simulink model "neural_network_based_adaptive_sliding"  (R2020b)
settings: Solver=ode45  StartTime=0  StopTime=10  RelTol=1e-3
settings Model: Creator=Melik  LastModifiedBy=asus
settings DataIOCC: ReturnWorkspaceOutputs=off
settings DebuggingCC: ArithmeticOperatorsInVariantConditions=warning
settings SFSimCC: SimUseLocalCustomCode=off  CustomCodeUndefinedFunction=UseInterfaceOnly
settings RTWCC: RTWUseLocalCustomCode=off

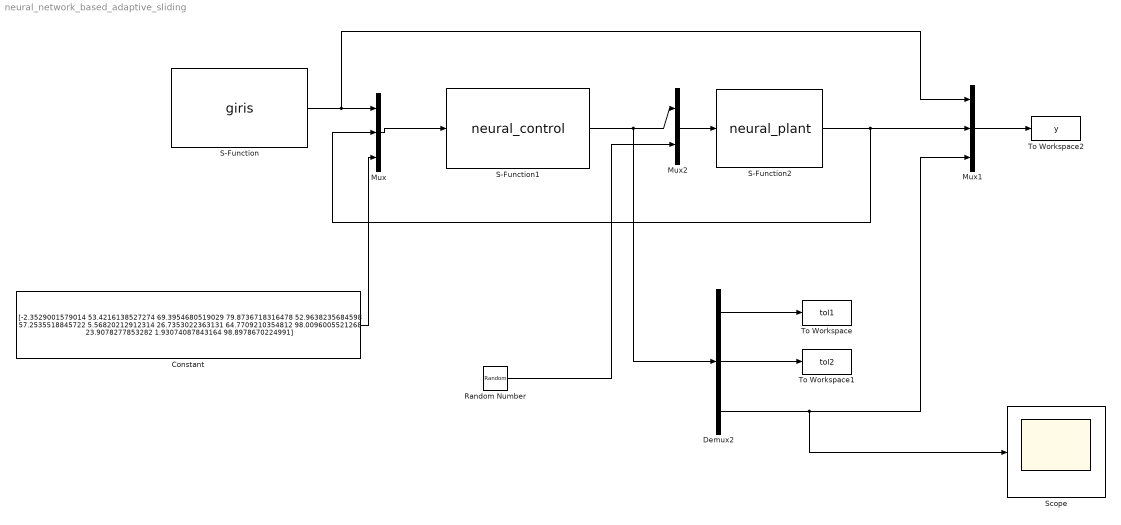
== system neural_network_based_adaptive_sliding ==
  Constant : Constant  Value=[-2.3529001579014 53.4216138527274 69.3954680519029 79.8736718316478 52.9638235684598 57.2535518845722 5.56820212912314 26.7353022363131 64.7709210354812 98.0096005521268 23.9078277853282 1.93074087843164 98.8978670224991]
  Demux2 : Demux  Outputs=3
  Mux : Mux  Inputs=3
  Mux1 : Mux  Inputs=3
  Mux2 : Mux  Inputs=2
  Random Number : RandomNumber  Variance=0.12  SampleTime=0.1
  S-Function : S-Function  FunctionName=giris  SFunctionDeploymentMode=off  EnableBusSupport=off
  S-Function1 : S-Function  FunctionName=neural_control  SFunctionDeploymentMode=off  EnableBusSupport=off
  S-Function2 : S-Function  FunctionName=neural_plant  SFunctionDeploymentMode=off  EnableBusSupport=off
  Scope : Scope
  To Workspace : ToWorkspace  VariableName=tol1  SaveFormat=Timeseries  SampleTime=-1
  To Workspace1 : ToWorkspace  VariableName=tol2  SaveFormat=Timeseries  SampleTime=-1
  To Workspace2 : ToWorkspace  VariableName=y  SaveFormat=Timeseries  SampleTime=-1
  wires:
  S-Function/1 -> Mux1/1, Mux/1
  Mux/1 -> S-Function1/1
  S-Function1/1 -> Demux2/1, Mux2/1
  S-Function2/1 -> Mux1/2, Mux/2
  Demux2/1 -> To Workspace/1
  Demux2/2 -> To Workspace1/1
  Demux2/3 -> Scope/1, Mux1/3
  Mux1/1 -> To Workspace2/1
  Random Number/1 -> Mux2/2
  Mux2/1 -> S-Function2/1
  Constant/1 -> Mux/3
